simulink model "simu_model"  (R2024b)
settings: Solver=VariableStepAuto  StartTime=0.0  StopTime=10.0  RelTol=1e-3
undefined symbols (not defined in the file or in its folder): SIM
settings Model: Creator=Leonardo Perina  LastModifiedBy=Leonardo Perina

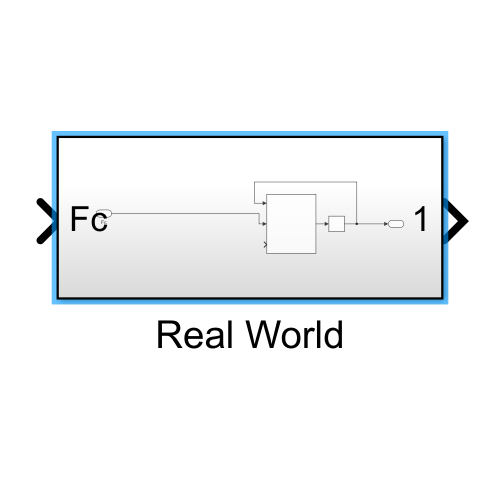
[thumbnail: Simulink's stored preview of the top-level diagram]
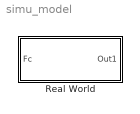
== system simu_model ==
  Real World : Subsystem

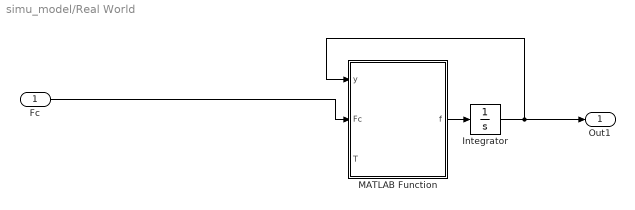
== system simu_model/Real World ==
  Fc : Inport
  Integrator : Integrator  InitialCondition=SIM.y0
  MATLAB Function : MATLAB Function  TreatAsAtomicUnit=on
  Out1 : Outport
  wires:
  Fc/1 -> MATLAB Function/2(Fc)
  MATLAB Function/1(f) -> Integrator/1
  Integrator/1 -> Out1/1, MATLAB Function/1(y)

== matlab function simu_model/Real World/MATLAB Function ==
  data: y input; f output; Fc input; T input
function f = fcn(y, Fc, T)

rho = AMB.rho;
g0  = AMB.g0;

% xp   = y(1);
vx   = y(2);
% yp   = y(3);
vy   = y(4);
th   = y(5);
thd  = y(6);
beta = atan2(vy,vx);
U2   = vx^2 + vy^2;
cl   = MSL.cl(th);
cd   = MSL.cd(th);


f = zeros(6, 1);

f(1) = vx;
f(3) = vy;
f(5) = thd;

Fa   = 0.5 * rho * U2 * MSL.l * MSL.diam;

f(2) = ( -Fc*sin( beta + th ) + T*cos( beta + th ) + ...
    Fa * (-cl*sin(beta) - cd*cos(beta))) * 1/MSL.m;
f(4) = (  Fc*cos( beta + th ) + T*sin( beta + th ) + ...
    Fa * (cl*cos(beta)  - cd*sin(beta))) * 1/MSL.m - g;
f(6) = (-Fc*MSL.lc - Fa*(cl*cos(th) + cd*sin(th))*MSL.la - MSL.thc*thd) * 1/MSL.J;


y = u;
